simulink model "LectureVersion"  (R2021b)
settings: Solver=VariableStepAuto  StartTime=0.0  StopTime=20  RelTol=1e-3
model workspace (MAT data in the model file):
  M_heater_air = 3600
  R_equivalent = 4.329e-07
  T_heater = 50
  Troom_IC = 20
  Var = 0
  c_air = 1005.4
  m_room_air = 1470
settings Model: Creator=jim  LastModifiedBy=jimd

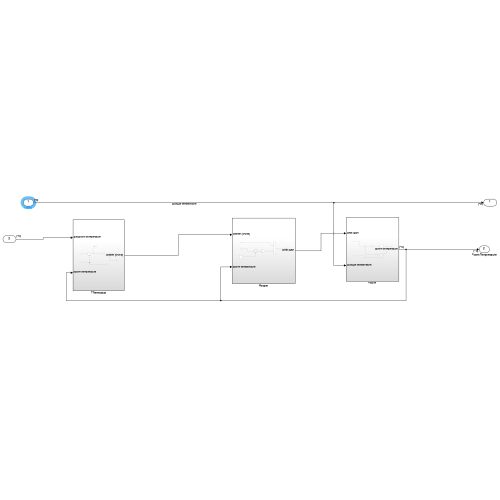
[thumbnail: Simulink's stored preview of the top-level diagram]
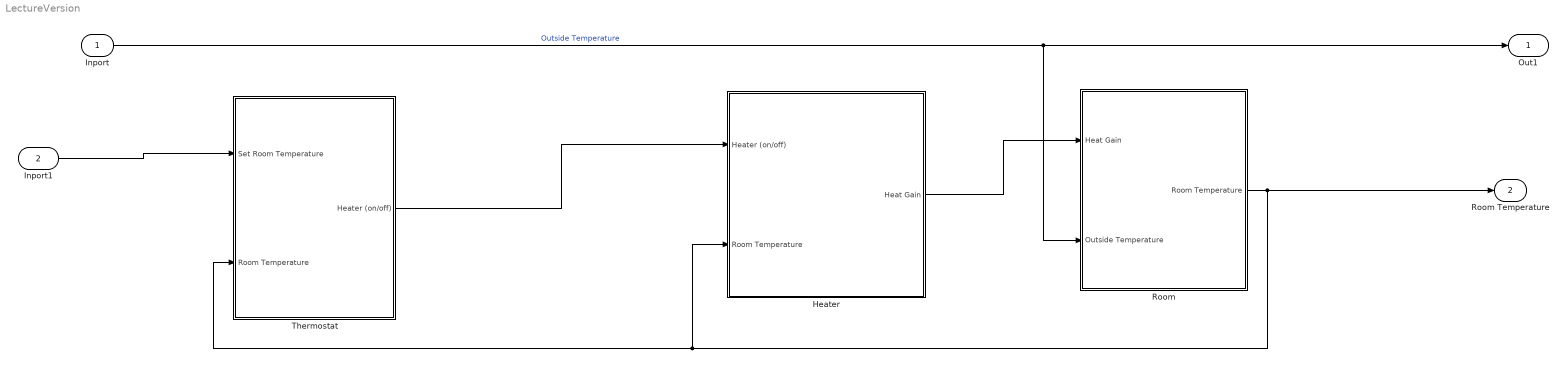
== system LectureVersion ==
  Inport : Inport  Unit=°C
  Inport1 : Inport  Port=2  Unit=°C
  Heater : Subsystem
  Room : Subsystem
  Thermostat : Subsystem
  Out1 : Outport  Unit=°C
  Room Temperature : Outport  Port=2  Unit=°C
  wires:
  Thermostat/1(Heater (on/off)) -> Heater/1(Heater (on/off))
  Room/1(Room Temperature) -> Heater/2(Room Temperature), Thermostat/2(Room Temperature), Room Temperature/1
  Heater/1(Heat Gain) -> Room/1(Heat Gain)
  Inport/1 -> Out1/1, Room/2(Outside Temperature)  "Outside Temperature"
  Inport1/1 -> Thermostat/1(Set Room Temperature)

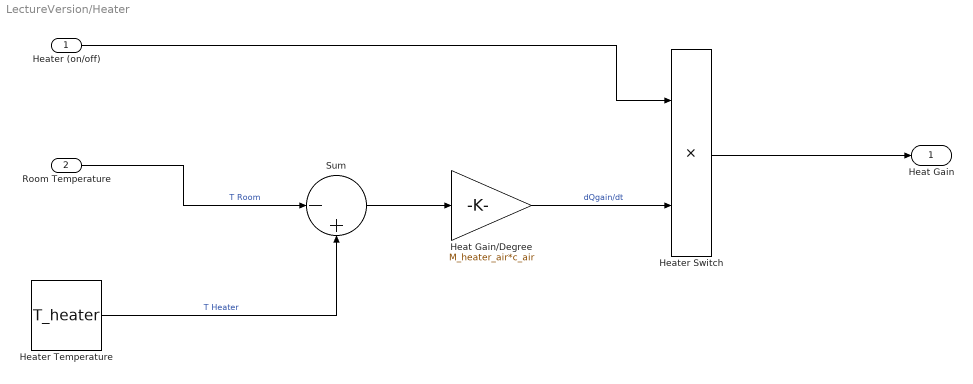
== system LectureVersion/Heater ==
  Heater (on/off) : Inport
  Room Temperature : Inport  Port=2
  Heat Gain/Degree : Gain  Gain=M_heater_air*c_air
  Heater Switch : Product
  Heater Temperature : Constant  Value=T_heater
  Sum : Sum  Inputs=|-+
  Heat Gain : Outport
  wires:
  Sum/1 -> Heat Gain/Degree/1
  Room Temperature/1 -> Sum/1  "T Room"
  Heater Temperature/1 -> Sum/2  "T Heater"
  Heater (on/off)/1 -> Heater Switch/1
  Heater Switch/1 -> Heat Gain/1
  Heat Gain/Degree/1 -> Heater Switch/2  "dQgain/dt"

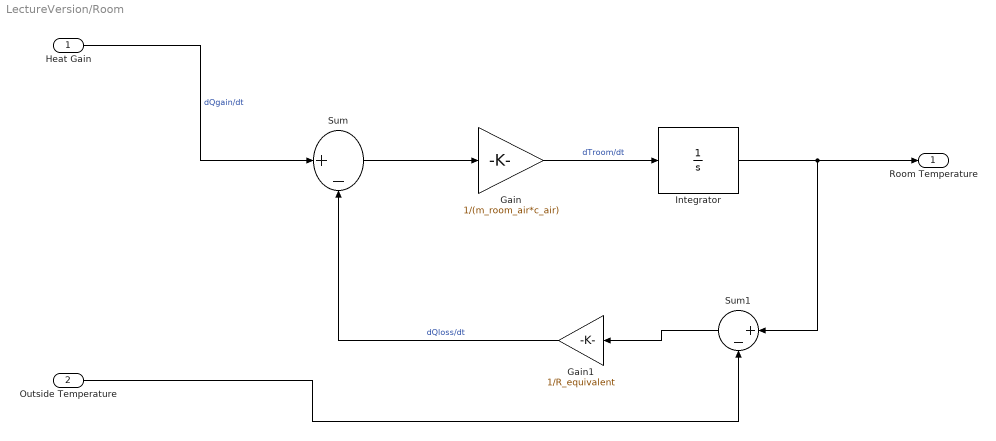
== system LectureVersion/Room ==
  Heat Gain : Inport
  Outside Temperature : Inport  Port=2
  Gain : Gain  Gain=1/(m_room_air*c_air)
  Gain1 : Gain  Gain=1/R_equivalent
  Integrator : Integrator  InitialCondition=Troom_IC
  Sum : Sum  Inputs=|+-
  Sum1 : Sum  Inputs=|+-
  Room Temperature : Outport
  wires:
  Heat Gain/1 -> Sum/1  "dQgain/dt"
  Sum/1 -> Gain/1
  Gain/1 -> Integrator/1  "dTroom/dt"
  Gain1/1 -> Sum/2  "dQloss/dt"
  Integrator/1 -> Sum1/1, Room Temperature/1
  Outside Temperature/1 -> Sum1/2
  Sum1/1 -> Gain1/1

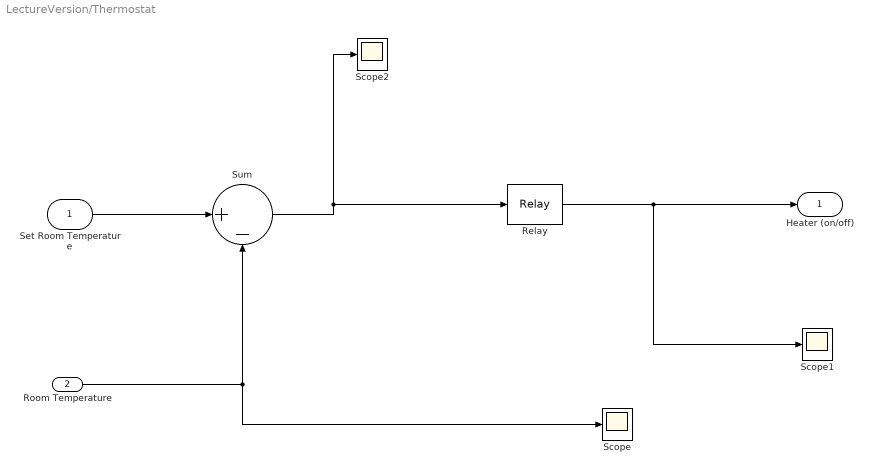
== system LectureVersion/Thermostat ==
  Set Room Temperature : Inport
  Room Temperature : Inport  Port=2
  Relay : Relay  OnSwitchValue=2  OffSwitchValue=-2
  Scope : Scope
  Scope1 : Scope
  Scope2 : Scope
  Sum : Sum  Inputs=|+-
  Heater (on/off) : Outport
  wires:
  Set Room Temperature/1 -> Sum/1
  Room Temperature/1 -> Sum/2, Scope/1
  Sum/1 -> Relay/1, Scope2/1
  Relay/1 -> Scope1/1, Heater (on/off)/1
